simulink model "ComparisonMod1Mod2Thev1Thev2ConstantTorque"  (R2019a)
settings: Solver=ode23t  StartTime=0.0  StopTime=3600  RelTol=1  AbsTol=1e-3  EnableMultiTasking=on
libraries: fl_lib x38, nesl_utility x26, ee_lib x4
settings Model: Creator=nikos  LastModifiedBy=nikos
settings DataIOCC: LimitDataPoints=on  SaveFormat=Array  ReturnWorkspaceOutputs=off
settings OptimizationCC: LifeSpan=inf
settings DebuggingCC: PregeneratedLibrarySubsystemCodeDiagnostic=none  SFUnexpectedBacktrackingDiag=warning  SFNoUnconditionalDefaultTransitionDiag=warning  SFExecutionAtInitializationDiag=none  ArithmeticOperatorsInVariantConditions=warning
settings HardwareCC: ProdBitPerPointer=32  ProdBitPerSizeT=32  ProdBitPerPtrDiffT=32  ProdLargestAtomicFloat=None  ProdIntDivRoundTo=Undefined  ProdEndianess=Unspecified  ProdWordSize=32  ProdHWDeviceType=32-bit Generic
settings ModelReferenceCC: PropagateSignalLabelsOutOfModel=off
settings SFSimCC: SimUseLocalCustomCode=off
settings RTWCC: RTWUseLocalCustomCode=off
settings CodeAppCC: StateflowObjectComments=on
settings GRTTargetCC: TargetLangStandard=C89/C90 (ANSI)  GeneratePreprocessorConditionals=Disable all
settings ConfigComp: CovMetricSettings=dw  CovHtmlReporting=on  CovSaveCumulativeToWorkspaceVar=on  CovSaveSingleToWorkspaceVar=on  CovExternalEMLEnable=off
settings SimscapeCC: SimscapeNormalizeSystem=off  SimscapeLogType=all  SimscapeLogDataHistory=10000

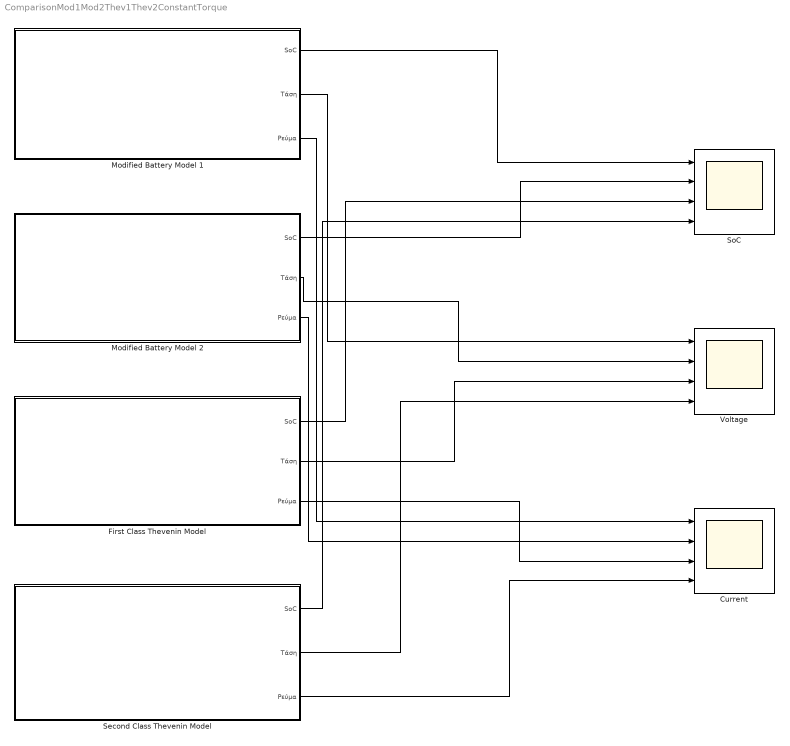
== system ComparisonMod1Mod2Thev1Thev2ConstantTorque ==
  Current : Scope  NumInputPorts=4
  First Class Thevenin Model : Subsystem
  Modified Battery Model 1 : Subsystem
  Modified Battery Model 2 : Subsystem
  "Second Class Thevenin Model " : Subsystem
  SoC : Scope  NumInputPorts=4
  Voltage : Scope  NumInputPorts=4
  wires:
  Modified Battery Model 1/1(SoC) -> SoC/1
  Modified Battery Model 2/1(SoC) -> SoC/2
  First Class Thevenin Model/1("SoC ") -> SoC/3
  "Second Class Thevenin Model "/1("SoC ") -> SoC/4
  Modified Battery Model 1/2(Τάση) -> Voltage/1
  Modified Battery Model 2/2(Τάση) -> Voltage/2
  First Class Thevenin Model/2(Τάση) -> Voltage/3
  "Second Class Thevenin Model "/2(Τάση) -> Voltage/4
  Modified Battery Model 1/3(Ρεύμα) -> Current/1
  Modified Battery Model 2/3(Ρεύμα) -> Current/2
  First Class Thevenin Model/3(Ρεύμα) -> Current/3
  "Second Class Thevenin Model "/3(Ρεύμα) -> Current/4

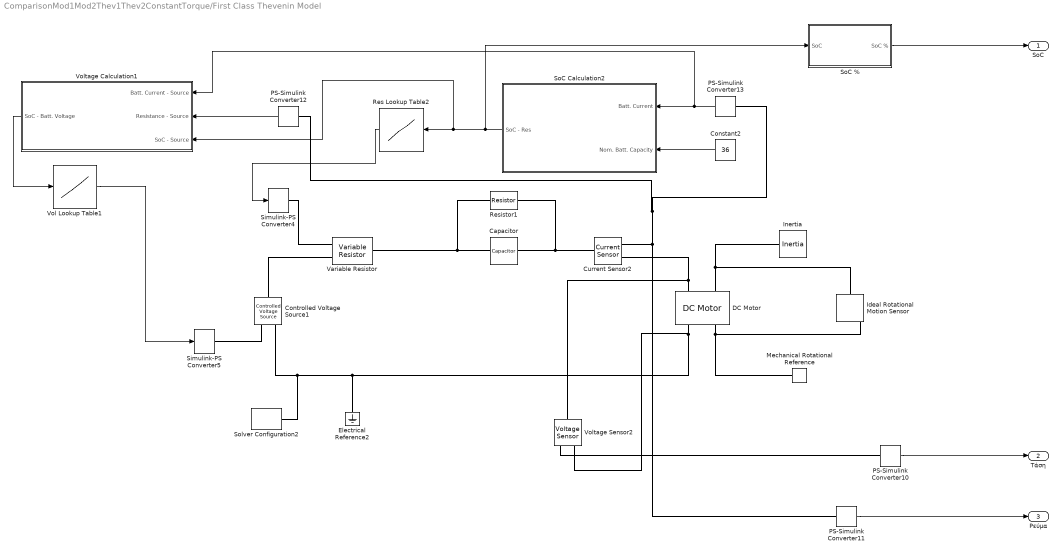
== system ComparisonMod1Mod2Thev1Thev2ConstantTorque/First Class Thevenin Model ==
  Capacitor : fl_lib/Electrical/Electrical Elements/Capacitor  c=1.5 F  r=1e-6 Ohm  g=0 1/Ohm  i_specify=off  i_priority=High  i=0 A  i_nominal_specify=off  i_nominal_unit=A  i_nominal_value=1  v_specify=off  v_priority=High  v=0 V  v_nominal_specify=off  v_nominal_unit=V  v_nominal_value=1  vc_specify=off  vc_priority=High  vc=0 V  vc_nominal_specify=off  vc_nominal_unit=V  vc_nominal_value=1
  Constant2 : Constant  Value=36
  Controlled Voltage Source1 : fl_lib/Electrical/Electrical Sources/Controlled Voltage Source
  Current Sensor2 : fl_lib/Electrical/Electrical Sensors/Current Sensor
  DC Motor : ee_lib/Electromechanical/Brushed Motors/DC Motor  parameterization=2  Ra=3.9 Ohm  La=12e-6 H  emf_or_torque=1  Kv=0.072e-3 V/rpm  Ki=6.876e-4 N*m/A  T_stall=240 mN*m  w_max=4300 rpm  w_rated=15000 rpm  P_rated=0.08 W  V_rated=14.7 V  J=0.01 g*cm^2  lam_param=2  lam=0 N*m/(rad/s)  i_noload=0.16 A  V_i_noload=1.5 V  speed0=0 rpm  alpha=3.93e-3 1/K  Tmeas=25 degC  thermal_mass=100 J/K  initial_temperature=25 degC
      settings: SourceProductName=Simscape Electrical
  Electrical Reference2 : fl_lib/Electrical/Electrical Elements/Electrical Reference
  Ideal Rotational Motion Sensor : fl_lib/Mechanical/Mechanical Sensors/Ideal Rotational Motion Sensor  offset=0 rad
  Inertia : fl_lib/Mechanical/Rotational Elements/Inertia  inertia=0.01 kg*m^2  w_specify=off  w_priority=High  w=0 rad/s  w_nominal_specify=off  w_nominal_unit=rad/s  w_nominal_value=1  t_specify=off  t_priority=None  t=0 N*m  t_nominal_specify=off  t_nominal_unit=N*m  t_nominal_value=1
  Mechanical Rotational Reference : fl_lib/Mechanical/Rotational Elements/Mechanical Rotational Reference
  PS-Simulink Converter{10..13} (4 alike) : nesl_utility/PS-Simulink Converter  PhysicalDomain=network_engine_domain  SubClassName=ps_output  LeftPortType=input  RightPortType=output  PseudoPeriodic=off  Frequencies=[]  Unit=1  AffineConversion=off
  Res Lookup Table2 : Lookup_n-D  NumberOfTableDimensions=1  BreakpointsForDimension1=[0, 10, 20, 30, 40, 50, 60, 70, 80, 90, 100]  Table=[0.011448, 0.011038, 0.011281, 0.011236, 0.010959, 0.010714, 0.010698, 0.010712, 0.010917, 0.011304, 0.011603]  InternalRulePriority=Speed  RndMeth=Simplest  InputSameDT=on
  Resistor1 : fl_lib/Electrical/Electrical Elements/Resistor  R=0.5 Ohm  i_specify=off  i_priority=High  i=0 A  i_nominal_specify=off  i_nominal_unit=A  i_nominal_value=1  v_specify=off  v_priority=High  v=0 V  v_nominal_specify=off  v_nominal_unit=V  v_nominal_value=1
  Simulink-PS Converter4 : nesl_utility/Simulink-PS Converter  PhysicalDomain=network_engine_domain  SubClassName=ps_input  LeftPortType=input  RightPortType=output  PseudoPeriodic=off  Frequencies=[]  NoiseDistribution=none  NoiseParameters=[]  Unit=1  AffineConversion=off  FilteringAndDerivatives=zero  SimscapeFilterOrder=1  InputFilterTimeConstant=0.001  UdotUserProvided=1
  Simulink-PS Converter5 : nesl_utility/Simulink-PS Converter  PhysicalDomain=network_engine_domain  SubClassName=ps_input  LeftPortType=input  RightPortType=output  PseudoPeriodic=off  Frequencies=[]  NoiseDistribution=none  NoiseParameters=[]  Unit=1  AffineConversion=off  FilteringAndDerivatives=filter  SimscapeFilterOrder=1  InputFilterTimeConstant=0.001  UdotUserProvided=1
  SoC % : Subsystem
  SoC Calculation2 : Subsystem
  Solver Configuration2 : nesl_utility/Solver Configuration  PhysicalDomain=network_engine_domain  SubClassName=solver  LeftPortType=input  RightPortType=generic  Tones=[]  Harmonics=[]  SimulateNoise=off  Profile=off  UseLocalSampling=off  EnableSwitchedLinearOptims=on  FrequencyDomain=off  UseCCode=off  RelTol=0.001  AbsTol=1e-06  MinStep=1e-09  ToWorkspace=off  RevertToSquareIcSolve=off  NumHomotopyIterations=100  PhasorMode=off  PhasorModeNumHarmonics=1  DoDC=off  ResidualTolerance=1e-09  UseLocalSolver=off  LocalSolverChoice=NE_BACKWARD_EULER_ADVANCER  LocalSolverSampleTime=0.001  DoFixedCost=off  MaxNonlinIter=3  MaxModeIter=2  LinearAlgebra=Sparse  EquationFormulation=NE_TIME_EF  DelaysMemoryBudget=1024  AutomaticFiltering=on  FilteringTimeConstant=0.001  PartitionStorageMethod=AS_NEEDED  PartitionMemoryBudget=1024  PartitionMethod=FAST
  Variable Resistor : fl_lib/Electrical/Electrical Elements/Variable Resistor  Rmin=0 Ohm  i_specify=off  i_priority=None  i=0 A  i_nominal_specify=off  i_nominal_unit=A  i_nominal_value=1  v_specify=off  v_priority=None  v=0 V  v_nominal_specify=off  v_nominal_unit=V  v_nominal_value=1
  Vol Lookup Table1 : Lookup_n-D  NumberOfTableDimensions=1  BreakpointsForDimension1=[0,10,20,30,40,50,60,70,80,90,100]  Table=[35.042,35.573,36.009,36.393,36.742,37.121,37.937,38.753,39.7,40.821,41.9299999]  InternalRulePriority=Speed  RndMeth=Simplest  InputSameDT=on
  Voltage Calculation1 : Subsystem
  Voltage Sensor2 : fl_lib/Electrical/Electrical Sensors/Voltage Sensor
  "SoC " : Outport
  Τάση : Outport  Port=2
  Ρεύμα : Outport  Port=3
  wires:
  PS-Simulink Converter12/1 -> Voltage Calculation1/2("Resistance - Source ")
  Voltage Calculation1/1("SoC - Batt. Voltage ") -> Vol Lookup Table1/1
  PS-Simulink Converter13/1 -> Voltage Calculation1/1(Batt. Current - Source), SoC Calculation2/1("Batt. Current ")
  PS-Simulink Converter10/1 -> Τάση/1
  Constant2/1 -> SoC Calculation2/2("Nom. Batt. Capacity ")
  SoC Calculation2/1(SoC - Res) -> SoC %/1(SoC), Res Lookup Table2/1, Voltage Calculation1/3(SoC - Source)
  Res Lookup Table2/1 -> Simulink-PS Converter4/1
  Vol Lookup Table1/1 -> Simulink-PS Converter5/1
  PS-Simulink Converter11/1 -> Ρεύμα/1
  SoC %/1(SoC %) -> "SoC "/1
  connections:
  Capacitor/RConn1 -- Resistor1/LConn1 -- Variable Resistor/RConn1
  PS-Simulink Converter13/LConn1 -- PS-Simulink Converter12/LConn1 -- PS-Simulink Converter11/LConn1 -- Current Sensor2/RConn1
  Voltage Sensor2/RConn2 -- DC Motor/RConn1 -- Electrical Reference2/LConn1 -- Controlled Voltage Source1/RConn2 -- Solver Configuration2/RConn1
  Simulink-PS Converter5/RConn1 -- Controlled Voltage Source1/RConn1
  Current Sensor2/RConn2 -- DC Motor/LConn1 -- Voltage Sensor2/LConn1
  Controlled Voltage Source1/LConn1 -- Variable Resistor/LConn2
  Voltage Sensor2/RConn1 -- PS-Simulink Converter10/LConn1
  Simulink-PS Converter4/RConn1 -- Variable Resistor/LConn1
  Capacitor/LConn1 -- Resistor1/RConn1 -- Current Sensor2/LConn1
  Inertia/LConn1 -- Ideal Rotational Motion Sensor/LConn1 -- DC Motor/LConn2
  Mechanical Rotational Reference/LConn1 -- Ideal Rotational Motion Sensor/RConn1 -- DC Motor/RConn2

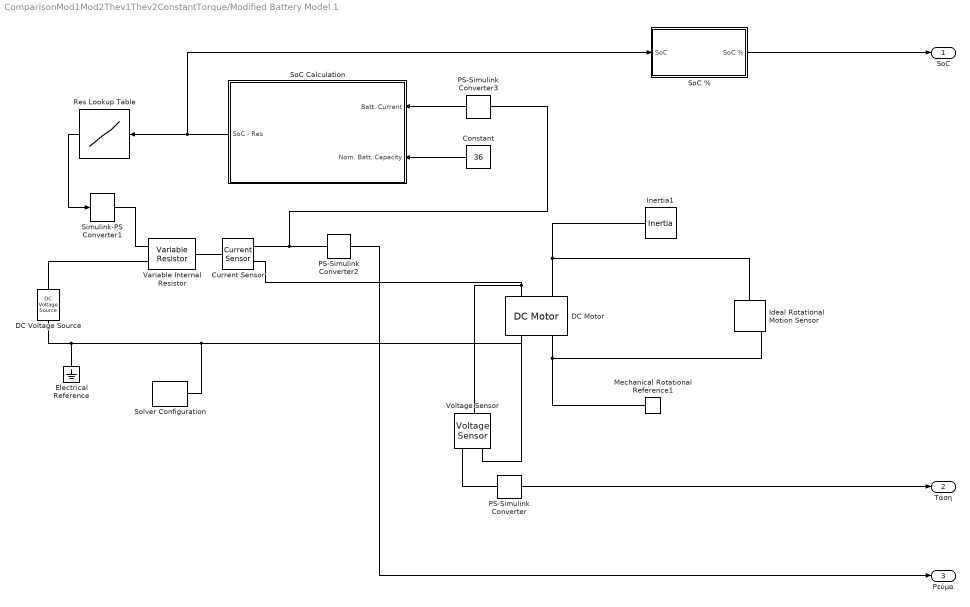
== system ComparisonMod1Mod2Thev1Thev2ConstantTorque/Modified Battery Model 1 ==
  Constant : Constant  Value=36
  Current Sensor : fl_lib/Electrical/Electrical Sensors/Current Sensor
  DC Motor : ee_lib/Electromechanical/Brushed Motors/DC Motor  parameterization=2  Ra=3.9 Ohm  La=12e-6 H  emf_or_torque=1  Kv=0.072e-3 V/rpm  Ki=6.876e-4 N*m/A  T_stall=240 mN*m  w_max=4300 rpm  w_rated=15000 rpm  P_rated=0.08 W  V_rated=14.7 V  J=0.01 g*cm^2  lam_param=2  lam=0 N*m/(rad/s)  i_noload=0.16 A  V_i_noload=1.5 V  speed0=0 rpm  alpha=3.93e-3 1/K  Tmeas=25 degC  thermal_mass=100 J/K  initial_temperature=25 degC
      settings: SourceProductName=Simscape Electrical
  DC Voltage Source : fl_lib/Electrical/Electrical Sources/DC Voltage Source  v0=72 V
  Electrical Reference : fl_lib/Electrical/Electrical Elements/Electrical Reference
  Ideal Rotational Motion Sensor : fl_lib/Mechanical/Mechanical Sensors/Ideal Rotational Motion Sensor  offset=0 rad
  Inertia1 : fl_lib/Mechanical/Rotational Elements/Inertia  inertia=0.01 kg*m^2  w_specify=off  w_priority=High  w=0 rad/s  w_nominal_specify=off  w_nominal_unit=rad/s  w_nominal_value=1  t_specify=off  t_priority=None  t=0 N*m  t_nominal_specify=off  t_nominal_unit=N*m  t_nominal_value=1
  Mechanical Rotational Reference1 : fl_lib/Mechanical/Rotational Elements/Mechanical Rotational Reference
  PS-Simulink Converter : nesl_utility/PS-Simulink Converter  PhysicalDomain=network_engine_domain  SubClassName=ps_output  LeftPortType=input  RightPortType=output  PseudoPeriodic=off  Frequencies=[]  Unit=1  AffineConversion=off
  PS-Simulink Converter2 : nesl_utility/PS-Simulink Converter  PhysicalDomain=network_engine_domain  SubClassName=ps_output  LeftPortType=input  RightPortType=output  PseudoPeriodic=off  Frequencies=[]  Unit=1  AffineConversion=off
  PS-Simulink Converter3 : nesl_utility/PS-Simulink Converter  PhysicalDomain=network_engine_domain  SubClassName=ps_output  LeftPortType=input  RightPortType=output  PseudoPeriodic=off  Frequencies=[]  Unit=1  AffineConversion=off
  Res Lookup Table : Lookup_n-D  NumberOfTableDimensions=1  BreakpointsForDimension1=[0, 10, 20, 30, 40, 50, 60, 70, 80, 90, 100]  Table=[0.011448, 0.011038, 0.011281, 0.011236, 0.010959, 0.010714, 0.010698, 0.010712, 0.010917, 0.011304, 0.011603]  InternalRulePriority=Speed  RndMeth=Simplest  InputSameDT=on
  Simulink-PS Converter1 : nesl_utility/Simulink-PS Converter  PhysicalDomain=network_engine_domain  SubClassName=ps_input  LeftPortType=input  RightPortType=output  PseudoPeriodic=off  Frequencies=[]  NoiseDistribution=none  NoiseParameters=[]  Unit=1  AffineConversion=off  FilteringAndDerivatives=zero  SimscapeFilterOrder=1  InputFilterTimeConstant=0.001  UdotUserProvided=1
  SoC % : Subsystem
  SoC Calculation : Subsystem
  Solver Configuration : nesl_utility/Solver Configuration  PhysicalDomain=network_engine_domain  SubClassName=solver  LeftPortType=input  RightPortType=generic  Tones=[]  Harmonics=[]  SimulateNoise=off  Profile=off  UseLocalSampling=off  EnableSwitchedLinearOptims=on  FrequencyDomain=off  UseCCode=off  RelTol=0.001  AbsTol=1e-06  MinStep=1e-09  ToWorkspace=off  RevertToSquareIcSolve=off  NumHomotopyIterations=100  PhasorMode=off  PhasorModeNumHarmonics=1  DoDC=off  ResidualTolerance=1e-09  UseLocalSolver=off  LocalSolverChoice=NE_BACKWARD_EULER_ADVANCER  LocalSolverSampleTime=0.001  DoFixedCost=off  MaxNonlinIter=3  MaxModeIter=2  LinearAlgebra=Sparse  EquationFormulation=NE_TIME_EF  DelaysMemoryBudget=1024  AutomaticFiltering=on  FilteringTimeConstant=0.001  PartitionStorageMethod=AS_NEEDED  PartitionMemoryBudget=1024  PartitionMethod=FAST
  Variable Internal Resistor : fl_lib/Electrical/Electrical Elements/Variable Resistor  Rmin=1 Ohm  i_specify=off  i_priority=High  i=0 A  i_nominal_specify=off  i_nominal_unit=A  i_nominal_value=1  v_specify=off  v_priority=High  v=0 V  v_nominal_specify=off  v_nominal_unit=V  v_nominal_value=1
  Voltage Sensor : fl_lib/Electrical/Electrical Sensors/Voltage Sensor
  SoC : Outport
  Τάση : Outport  Port=2
  Ρεύμα : Outport  Port=3
  wires:
  SoC Calculation/1(SoC - Res) -> SoC %/1(SoC), Res Lookup Table/1
  PS-Simulink Converter2/1 -> Ρεύμα/1
  Constant/1 -> SoC Calculation/2("Nom. Batt. Capacity ")
  Res Lookup Table/1 -> Simulink-PS Converter1/1
  PS-Simulink Converter3/1 -> SoC Calculation/1("Batt. Current ")
  PS-Simulink Converter/1 -> Τάση/1
  SoC %/1(SoC %) -> SoC/1
  connections:
  PS-Simulink Converter/LConn1 -- Voltage Sensor/RConn1
  Current Sensor/LConn1 -- Variable Internal Resistor/RConn1
  DC Voltage Source/LConn1 -- Variable Internal Resistor/LConn2
  DC Voltage Source/RConn1 -- DC Motor/RConn1 -- Voltage Sensor/RConn2 -- Solver Configuration/RConn1 -- Electrical Reference/LConn1
  Voltage Sensor/LConn1 -- DC Motor/LConn1 -- Current Sensor/RConn2
  PS-Simulink Converter2/LConn1 -- Current Sensor/RConn1 -- PS-Simulink Converter3/LConn1
  Simulink-PS Converter1/RConn1 -- Variable Internal Resistor/LConn1
  DC Motor/LConn2 -- Ideal Rotational Motion Sensor/LConn1 -- Inertia1/LConn1
  DC Motor/RConn2 -- Ideal Rotational Motion Sensor/RConn1 -- Mechanical Rotational Reference1/LConn1

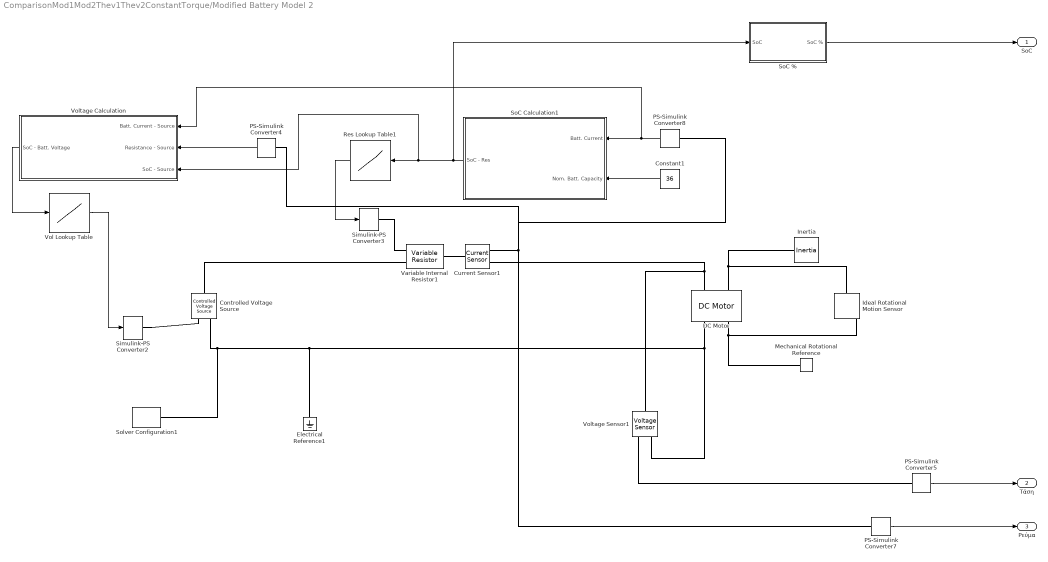
== system ComparisonMod1Mod2Thev1Thev2ConstantTorque/Modified Battery Model 2 ==
  Constant1 : Constant  Value=36
  Controlled Voltage Source : fl_lib/Electrical/Electrical Sources/Controlled Voltage Source
  Current Sensor1 : fl_lib/Electrical/Electrical Sensors/Current Sensor
  DC Motor : ee_lib/Electromechanical/Brushed Motors/DC Motor  parameterization=2  Ra=3.9 Ohm  La=12e-6 H  emf_or_torque=1  Kv=0.072e-3 V/rpm  Ki=6.876e-4 N*m/A  T_stall=240 mN*m  w_max=4300 rpm  w_rated=15000 rpm  P_rated=0.08 W  V_rated=14.7 V  J=0.01 g*cm^2  lam_param=2  lam=0 N*m/(rad/s)  i_noload=0.16 A  V_i_noload=1.5 V  speed0=0 rpm  alpha=3.93e-3 1/K  Tmeas=25 degC  thermal_mass=100 J/K  initial_temperature=25 degC
      settings: SourceProductName=Simscape Electrical
  Electrical Reference1 : fl_lib/Electrical/Electrical Elements/Electrical Reference
  Ideal Rotational Motion Sensor : fl_lib/Mechanical/Mechanical Sensors/Ideal Rotational Motion Sensor  offset=0 rad
  Inertia : fl_lib/Mechanical/Rotational Elements/Inertia  inertia=0.01 kg*m^2  w_specify=off  w_priority=High  w=0 rad/s  w_nominal_specify=off  w_nominal_unit=rad/s  w_nominal_value=1  t_specify=off  t_priority=None  t=0 N*m  t_nominal_specify=off  t_nominal_unit=N*m  t_nominal_value=1
  Mechanical Rotational Reference : fl_lib/Mechanical/Rotational Elements/Mechanical Rotational Reference
  PS-Simulink Converter{4..5,7..8} (4 alike) : nesl_utility/PS-Simulink Converter  PhysicalDomain=network_engine_domain  SubClassName=ps_output  LeftPortType=input  RightPortType=output  PseudoPeriodic=off  Frequencies=[]  Unit=1  AffineConversion=off
  Res Lookup Table1 : Lookup_n-D  NumberOfTableDimensions=1  BreakpointsForDimension1=[0, 10, 20, 30, 40, 50, 60, 70, 80, 90, 100]  Table=[0.011448, 0.011038, 0.011281, 0.011236, 0.010959, 0.010714, 0.010698, 0.010712, 0.010917, 0.011304, 0.011603]  InternalRulePriority=Speed  RndMeth=Simplest  InputSameDT=on
  Simulink-PS Converter2 : nesl_utility/Simulink-PS Converter  PhysicalDomain=network_engine_domain  SubClassName=ps_input  LeftPortType=input  RightPortType=output  PseudoPeriodic=off  Frequencies=[]  NoiseDistribution=none  NoiseParameters=[]  Unit=1  AffineConversion=off  FilteringAndDerivatives=filter  SimscapeFilterOrder=1  InputFilterTimeConstant=0.001  UdotUserProvided=1
  Simulink-PS Converter3 : nesl_utility/Simulink-PS Converter  PhysicalDomain=network_engine_domain  SubClassName=ps_input  LeftPortType=input  RightPortType=output  PseudoPeriodic=off  Frequencies=[]  NoiseDistribution=none  NoiseParameters=[]  Unit=1  AffineConversion=off  FilteringAndDerivatives=zero  SimscapeFilterOrder=1  InputFilterTimeConstant=0.001  UdotUserProvided=1
  SoC % : Subsystem
  SoC Calculation1 : Subsystem
  Solver Configuration1 : nesl_utility/Solver Configuration  PhysicalDomain=network_engine_domain  SubClassName=solver  LeftPortType=input  RightPortType=generic  Tones=[]  Harmonics=[]  SimulateNoise=off  Profile=off  UseLocalSampling=off  EnableSwitchedLinearOptims=on  FrequencyDomain=off  UseCCode=off  RelTol=0.001  AbsTol=1e-06  MinStep=1e-09  ToWorkspace=off  RevertToSquareIcSolve=off  NumHomotopyIterations=100  PhasorMode=off  PhasorModeNumHarmonics=1  DoDC=off  ResidualTolerance=1e-09  UseLocalSolver=off  LocalSolverChoice=NE_BACKWARD_EULER_ADVANCER  LocalSolverSampleTime=0.001  DoFixedCost=off  MaxNonlinIter=3  MaxModeIter=2  LinearAlgebra=Sparse  EquationFormulation=NE_TIME_EF  DelaysMemoryBudget=1024  AutomaticFiltering=on  FilteringTimeConstant=0.001  PartitionStorageMethod=AS_NEEDED  PartitionMemoryBudget=1024  PartitionMethod=FAST
  Variable Internal Resistor1 : fl_lib/Electrical/Electrical Elements/Variable Resistor  Rmin=1 Ohm  i_specify=off  i_priority=High  i=0 A  i_nominal_specify=off  i_nominal_unit=A  i_nominal_value=1  v_specify=off  v_priority=High  v=0 V  v_nominal_specify=off  v_nominal_unit=V  v_nominal_value=1
  Vol Lookup Table : Lookup_n-D  NumberOfTableDimensions=1  BreakpointsForDimension1=[0,10,20,30,40,50,60,70,80,90,100]  Table=[35.042,35.573,36.009,36.393,36.742,37.121,37.937,38.753,39.7,40.821,41.9299999]  InternalRulePriority=Speed  RndMeth=Simplest  InputSameDT=on
  Voltage Calculation : Subsystem
  Voltage Sensor1 : fl_lib/Electrical/Electrical Sensors/Voltage Sensor
  SoC : Outport
  Τάση : Outport  Port=2
  Ρεύμα : Outport  Port=3
  wires:
  Res Lookup Table1/1 -> Simulink-PS Converter3/1
  PS-Simulink Converter5/1 -> Τάση/1
  SoC Calculation1/1(SoC - Res) -> SoC %/1(SoC), Res Lookup Table1/1, Voltage Calculation/3(SoC - Source)
  PS-Simulink Converter8/1 -> SoC Calculation1/1("Batt. Current "), Voltage Calculation/1(Batt. Current - Source)
  PS-Simulink Converter4/1 -> Voltage Calculation/2("Resistance - Source ")
  Constant1/1 -> SoC Calculation1/2("Nom. Batt. Capacity ")
  PS-Simulink Converter7/1 -> Ρεύμα/1
  Voltage Calculation/1("SoC - Batt. Voltage ") -> Vol Lookup Table/1
  Vol Lookup Table/1 -> Simulink-PS Converter2/1
  SoC %/1(SoC %) -> SoC/1
  connections:
  Controlled Voltage Source/RConn2 -- Electrical Reference1/LConn1 -- DC Motor/RConn1 -- Voltage Sensor1/RConn2 -- Solver Configuration1/RConn1
  Current Sensor1/RConn2 -- DC Motor/LConn1 -- Voltage Sensor1/LConn1
  PS-Simulink Converter7/LConn1 -- Current Sensor1/RConn1 -- PS-Simulink Converter8/LConn1 -- PS-Simulink Converter4/LConn1
  Simulink-PS Converter3/RConn1 -- Variable Internal Resistor1/LConn1
  Simulink-PS Converter2/RConn1 -- Controlled Voltage Source/RConn1
  PS-Simulink Converter5/LConn1 -- Voltage Sensor1/RConn1
  Current Sensor1/LConn1 -- Variable Internal Resistor1/RConn1
  Controlled Voltage Source/LConn1 -- Variable Internal Resistor1/LConn2
  DC Motor/LConn2 -- Ideal Rotational Motion Sensor/LConn1 -- Inertia/LConn1
  DC Motor/RConn2 -- Ideal Rotational Motion Sensor/RConn1 -- Mechanical Rotational Reference/LConn1

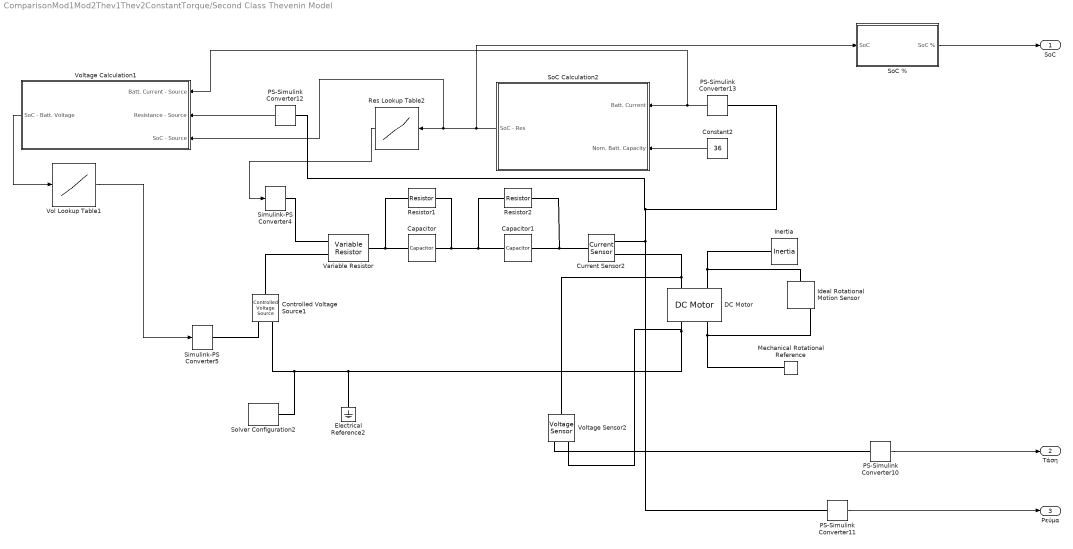
== system ComparisonMod1Mod2Thev1Thev2ConstantTorque/Second Class Thevenin Model  ==
  Capacitor : fl_lib/Electrical/Electrical Elements/Capacitor  c=1.5 F  r=1e-6 Ohm  g=0 1/Ohm  i_specify=off  i_priority=High  i=0 A  i_nominal_specify=off  i_nominal_unit=A  i_nominal_value=1  v_specify=off  v_priority=High  v=0 V  v_nominal_specify=off  v_nominal_unit=V  v_nominal_value=1  vc_specify=off  vc_priority=High  vc=0 V  vc_nominal_specify=off  vc_nominal_unit=V  vc_nominal_value=1
  Capacitor1 : fl_lib/Electrical/Electrical Elements/Capacitor  c=1.5 F  r=1e-6 Ohm  g=0 1/Ohm  i_specify=off  i_priority=High  i=0 A  i_nominal_specify=off  i_nominal_unit=A  i_nominal_value=1  v_specify=off  v_priority=High  v=0 V  v_nominal_specify=off  v_nominal_unit=V  v_nominal_value=1  vc_specify=off  vc_priority=High  vc=0 V  vc_nominal_specify=off  vc_nominal_unit=V  vc_nominal_value=1
  Constant2 : Constant  Value=36
  Controlled Voltage Source1 : fl_lib/Electrical/Electrical Sources/Controlled Voltage Source
  Current Sensor2 : fl_lib/Electrical/Electrical Sensors/Current Sensor
  DC Motor : ee_lib/Electromechanical/Brushed Motors/DC Motor  parameterization=2  Ra=3.9 Ohm  La=12e-6 H  emf_or_torque=1  Kv=0.072e-3 V/rpm  Ki=6.876e-4 N*m/A  T_stall=240 mN*m  w_max=4300 rpm  w_rated=15000 rpm  P_rated=0.08 W  V_rated=14.7 V  J=0.01 g*cm^2  lam_param=2  lam=0 N*m/(rad/s)  i_noload=0.16 A  V_i_noload=1.5 V  speed0=0 rpm  alpha=3.93e-3 1/K  Tmeas=25 degC  thermal_mass=100 J/K  initial_temperature=25 degC
      settings: SourceProductName=Simscape Electrical
  Electrical Reference2 : fl_lib/Electrical/Electrical Elements/Electrical Reference
  Ideal Rotational Motion Sensor : fl_lib/Mechanical/Mechanical Sensors/Ideal Rotational Motion Sensor  offset=0 rad
  Inertia : fl_lib/Mechanical/Rotational Elements/Inertia  inertia=0.01 kg*m^2  w_specify=off  w_priority=High  w=0 rad/s  w_nominal_specify=off  w_nominal_unit=rad/s  w_nominal_value=1  t_specify=off  t_priority=None  t=0 N*m  t_nominal_specify=off  t_nominal_unit=N*m  t_nominal_value=1
  Mechanical Rotational Reference : fl_lib/Mechanical/Rotational Elements/Mechanical Rotational Reference
  PS-Simulink Converter{10..13} (4 alike) : nesl_utility/PS-Simulink Converter  PhysicalDomain=network_engine_domain  SubClassName=ps_output  LeftPortType=input  RightPortType=output  PseudoPeriodic=off  Frequencies=[]  Unit=1  AffineConversion=off
  Res Lookup Table2 : Lookup_n-D  NumberOfTableDimensions=1  BreakpointsForDimension1=[0, 10, 20, 30, 40, 50, 60, 70, 80, 90, 100]  Table=[0.011448, 0.011038, 0.011281, 0.011236, 0.010959, 0.010714, 0.010698, 0.010712, 0.010917, 0.011304, 0.011603]  InternalRulePriority=Speed  RndMeth=Simplest  InputSameDT=on
  Resistor1 : fl_lib/Electrical/Electrical Elements/Resistor  R=0.5 Ohm  i_specify=off  i_priority=High  i=0 A  i_nominal_specify=off  i_nominal_unit=A  i_nominal_value=1  v_specify=off  v_priority=High  v=0 V  v_nominal_specify=off  v_nominal_unit=V  v_nominal_value=1
  Resistor2 : fl_lib/Electrical/Electrical Elements/Resistor  R=0.5 Ohm  i_specify=off  i_priority=High  i=0 A  i_nominal_specify=off  i_nominal_unit=A  i_nominal_value=1  v_specify=off  v_priority=High  v=0 V  v_nominal_specify=off  v_nominal_unit=V  v_nominal_value=1
  Simulink-PS Converter4 : nesl_utility/Simulink-PS Converter  PhysicalDomain=network_engine_domain  SubClassName=ps_input  LeftPortType=input  RightPortType=output  PseudoPeriodic=off  Frequencies=[]  NoiseDistribution=none  NoiseParameters=[]  Unit=1  AffineConversion=off  FilteringAndDerivatives=zero  SimscapeFilterOrder=1  InputFilterTimeConstant=0.001  UdotUserProvided=1
  Simulink-PS Converter5 : nesl_utility/Simulink-PS Converter  PhysicalDomain=network_engine_domain  SubClassName=ps_input  LeftPortType=input  RightPortType=output  PseudoPeriodic=off  Frequencies=[]  NoiseDistribution=none  NoiseParameters=[]  Unit=1  AffineConversion=off  FilteringAndDerivatives=filter  SimscapeFilterOrder=1  InputFilterTimeConstant=0.001  UdotUserProvided=1
  SoC % : Subsystem
  SoC Calculation2 : Subsystem
  Solver Configuration2 : nesl_utility/Solver Configuration  PhysicalDomain=network_engine_domain  SubClassName=solver  LeftPortType=input  RightPortType=generic  Tones=[]  Harmonics=[]  SimulateNoise=off  Profile=off  UseLocalSampling=off  EnableSwitchedLinearOptims=on  FrequencyDomain=off  UseCCode=off  RelTol=0.001  AbsTol=1e-06  MinStep=1e-09  ToWorkspace=off  RevertToSquareIcSolve=off  NumHomotopyIterations=100  PhasorMode=off  PhasorModeNumHarmonics=1  DoDC=off  ResidualTolerance=1e-09  UseLocalSolver=off  LocalSolverChoice=NE_BACKWARD_EULER_ADVANCER  LocalSolverSampleTime=0.001  DoFixedCost=off  MaxNonlinIter=3  MaxModeIter=2  LinearAlgebra=Sparse  EquationFormulation=NE_TIME_EF  DelaysMemoryBudget=1024  AutomaticFiltering=on  FilteringTimeConstant=0.001  PartitionStorageMethod=AS_NEEDED  PartitionMemoryBudget=1024  PartitionMethod=FAST
  Variable Resistor : fl_lib/Electrical/Electrical Elements/Variable Resistor  Rmin=0 Ohm  i_specify=off  i_priority=None  i=0 A  i_nominal_specify=off  i_nominal_unit=A  i_nominal_value=1  v_specify=off  v_priority=None  v=0 V  v_nominal_specify=off  v_nominal_unit=V  v_nominal_value=1
  Vol Lookup Table1 : Lookup_n-D  NumberOfTableDimensions=1  BreakpointsForDimension1=[0,10,20,30,40,50,60,70,80,90,100]  Table=[35.042,35.573,36.009,36.393,36.742,37.121,37.937,38.753,39.7,40.821,41.9299999]  InternalRulePriority=Speed  RndMeth=Simplest  InputSameDT=on
  Voltage Calculation1 : Subsystem
  Voltage Sensor2 : fl_lib/Electrical/Electrical Sensors/Voltage Sensor
  "SoC " : Outport
  Τάση : Outport  Port=2
  Ρεύμα : Outport  Port=3
  wires:
  PS-Simulink Converter13/1 -> Voltage Calculation1/1(Batt. Current - Source), SoC Calculation2/1("Batt. Current ")
  SoC Calculation2/1(SoC - Res) -> SoC %/1(SoC), Res Lookup Table2/1, Voltage Calculation1/3(SoC - Source)
  PS-Simulink Converter11/1 -> Ρεύμα/1
  PS-Simulink Converter12/1 -> Voltage Calculation1/2("Resistance - Source ")
  PS-Simulink Converter10/1 -> Τάση/1
  Constant2/1 -> SoC Calculation2/2("Nom. Batt. Capacity ")
  Res Lookup Table2/1 -> Simulink-PS Converter4/1
  Vol Lookup Table1/1 -> Simulink-PS Converter5/1
  Voltage Calculation1/1("SoC - Batt. Voltage ") -> Vol Lookup Table1/1
  SoC %/1(SoC %) -> "SoC "/1
  connections:
  Voltage Sensor2/RConn1 -- PS-Simulink Converter10/LConn1
  Controlled Voltage Source1/LConn1 -- Variable Resistor/LConn2
  Capacitor/LConn1 -- Resistor2/LConn1 -- Capacitor1/RConn1 -- Resistor1/RConn1
  Solver Configuration2/RConn1 -- Voltage Sensor2/RConn2 -- DC Motor/RConn1 -- Electrical Reference2/LConn1 -- Controlled Voltage Source1/RConn2
  Simulink-PS Converter5/RConn1 -- Controlled Voltage Source1/RConn1
  Capacitor1/LConn1 -- Resistor2/RConn1 -- Current Sensor2/LConn1
  Current Sensor2/RConn2 -- DC Motor/LConn1 -- Voltage Sensor2/LConn1
  PS-Simulink Converter13/LConn1 -- PS-Simulink Converter11/LConn1 -- Current Sensor2/RConn1 -- PS-Simulink Converter12/LConn1
  Capacitor/RConn1 -- Resistor1/LConn1 -- Variable Resistor/RConn1
  Simulink-PS Converter4/RConn1 -- Variable Resistor/LConn1
  Inertia/LConn1 -- Ideal Rotational Motion Sensor/LConn1 -- DC Motor/LConn2
  Mechanical Rotational Reference/LConn1 -- Ideal Rotational Motion Sensor/RConn1 -- DC Motor/RConn2

== system ComparisonMod1Mod2Thev1Thev2ConstantTorque/First Class Thevenin Model/SoC % ==
  SoC : Inport
  Gain : Gain  Gain=1/36
  Gain1 : Gain  Gain=100
  SoC % : Outport
  wires:
  Gain/1 -> Gain1/1
  SoC/1 -> Gain/1
  Gain1/1 -> SoC %/1

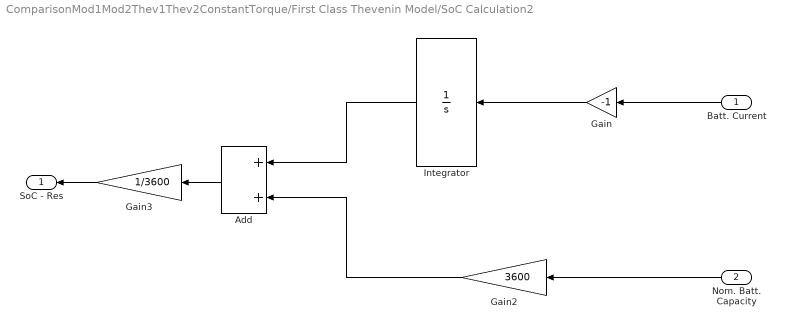
== system ComparisonMod1Mod2Thev1Thev2ConstantTorque/First Class Thevenin Model/SoC Calculation2 ==
  "Batt. Current " : Inport
  "Nom. Batt. Capacity " : Inport  Port=2  OutMin=0  OutMax=100
  Add : Sum
  Gain : Gain  Gain=-1
  Gain2 : Gain  Gain=3600
  Gain3 : Gain  Gain=1/3600
  Integrator : Integrator
  SoC - Res : Outport
  wires:
  Gain3/1 -> SoC - Res/1
  Integrator/1 -> Add/1
  Add/1 -> Gain3/1
  Gain2/1 -> Add/2
  "Nom. Batt. Capacity "/1 -> Gain2/1
  Gain/1 -> Integrator/1
  "Batt. Current "/1 -> Gain/1

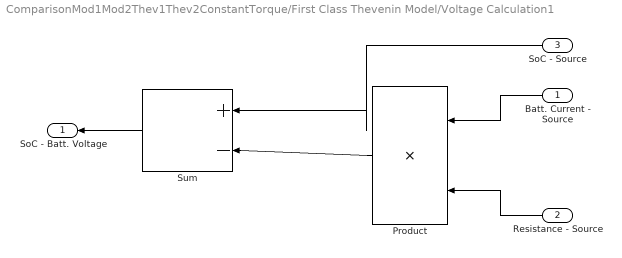
== system ComparisonMod1Mod2Thev1Thev2ConstantTorque/First Class Thevenin Model/Voltage Calculation1 ==
  Batt. Current - Source : Inport
  "Resistance - Source " : Inport  Port=2
  SoC - Source : Inport  Port=3
  Product : Product
  Sum : Sum  Inputs=|+-
  "SoC - Batt. Voltage " : Outport
  wires:
  Product/1 -> Sum/2
  Batt. Current - Source/1 -> Product/1
  "Resistance - Source "/1 -> Product/2
  SoC - Source/1 -> Sum/1
  Sum/1 -> "SoC - Batt. Voltage "/1

== system ComparisonMod1Mod2Thev1Thev2ConstantTorque/Modified Battery Model 1/SoC % ==
  SoC : Inport
  Gain : Gain  Gain=1/36
  Gain1 : Gain  Gain=100
  SoC % : Outport
  wires:
  Gain/1 -> Gain1/1
  SoC/1 -> Gain/1
  Gain1/1 -> SoC %/1

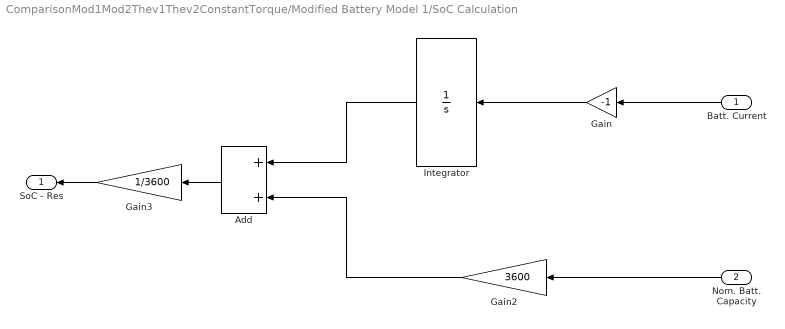
== system ComparisonMod1Mod2Thev1Thev2ConstantTorque/Modified Battery Model 1/SoC Calculation ==
  "Batt. Current " : Inport
  "Nom. Batt. Capacity " : Inport  Port=2  OutMin=0  OutMax=100
  Add : Sum
  Gain : Gain  Gain=-1
  Gain2 : Gain  Gain=3600
  Gain3 : Gain  Gain=1/3600
  Integrator : Integrator
  SoC - Res : Outport
  wires:
  "Batt. Current "/1 -> Gain/1
  Gain/1 -> Integrator/1
  "Nom. Batt. Capacity "/1 -> Gain2/1
  Gain2/1 -> Add/2
  Add/1 -> Gain3/1
  Integrator/1 -> Add/1
  Gain3/1 -> SoC - Res/1

== system ComparisonMod1Mod2Thev1Thev2ConstantTorque/Modified Battery Model 2/SoC % ==
  SoC : Inport
  Gain : Gain  Gain=1/36
  Gain1 : Gain  Gain=100
  SoC % : Outport
  wires:
  Gain/1 -> Gain1/1
  SoC/1 -> Gain/1
  Gain1/1 -> SoC %/1

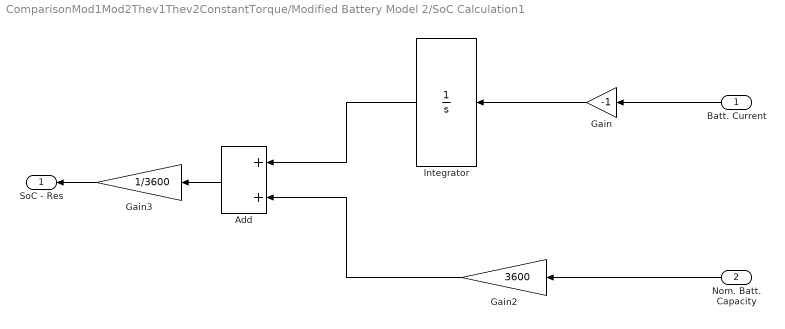
== system ComparisonMod1Mod2Thev1Thev2ConstantTorque/Modified Battery Model 2/SoC Calculation1 ==
  "Batt. Current " : Inport
  "Nom. Batt. Capacity " : Inport  Port=2  OutMin=0  OutMax=100
  Add : Sum
  Gain : Gain  Gain=-1
  Gain2 : Gain  Gain=3600
  Gain3 : Gain  Gain=1/3600
  Integrator : Integrator
  SoC - Res : Outport
  wires:
  "Batt. Current "/1 -> Gain/1
  Gain/1 -> Integrator/1
  "Nom. Batt. Capacity "/1 -> Gain2/1
  Gain2/1 -> Add/2
  Add/1 -> Gain3/1
  Integrator/1 -> Add/1
  Gain3/1 -> SoC - Res/1

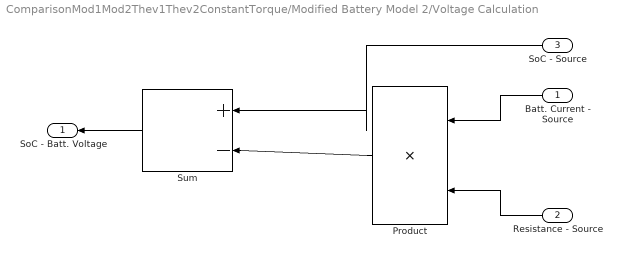
== system ComparisonMod1Mod2Thev1Thev2ConstantTorque/Modified Battery Model 2/Voltage Calculation ==
  Batt. Current - Source : Inport
  "Resistance - Source " : Inport  Port=2
  SoC - Source : Inport  Port=3
  Product : Product
  Sum : Sum  Inputs=|+-
  "SoC - Batt. Voltage " : Outport
  wires:
  Sum/1 -> "SoC - Batt. Voltage "/1
  SoC - Source/1 -> Sum/1
  "Resistance - Source "/1 -> Product/2
  Batt. Current - Source/1 -> Product/1
  Product/1 -> Sum/2

== system ComparisonMod1Mod2Thev1Thev2ConstantTorque/Second Class Thevenin Model /SoC % ==
  SoC : Inport
  Gain : Gain  Gain=1/36
  Gain1 : Gain  Gain=100
  SoC % : Outport
  wires:
  Gain/1 -> Gain1/1
  SoC/1 -> Gain/1
  Gain1/1 -> SoC %/1

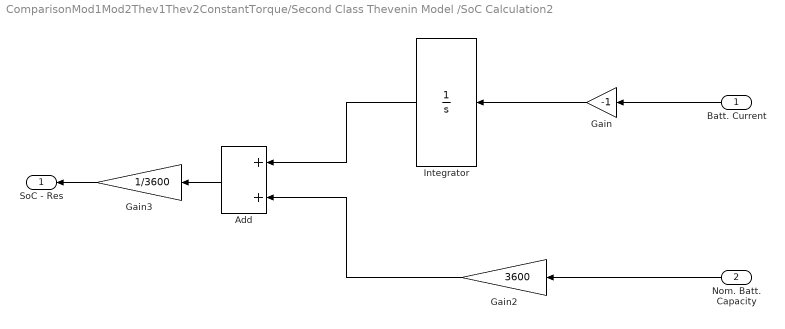
== system ComparisonMod1Mod2Thev1Thev2ConstantTorque/Second Class Thevenin Model /SoC Calculation2 ==
  "Batt. Current " : Inport
  "Nom. Batt. Capacity " : Inport  Port=2  OutMin=0  OutMax=100
  Add : Sum
  Gain : Gain  Gain=-1
  Gain2 : Gain  Gain=3600
  Gain3 : Gain  Gain=1/3600
  Integrator : Integrator
  SoC - Res : Outport
  wires:
  Gain3/1 -> SoC - Res/1
  Integrator/1 -> Add/1
  Add/1 -> Gain3/1
  Gain2/1 -> Add/2
  "Nom. Batt. Capacity "/1 -> Gain2/1
  Gain/1 -> Integrator/1
  "Batt. Current "/1 -> Gain/1

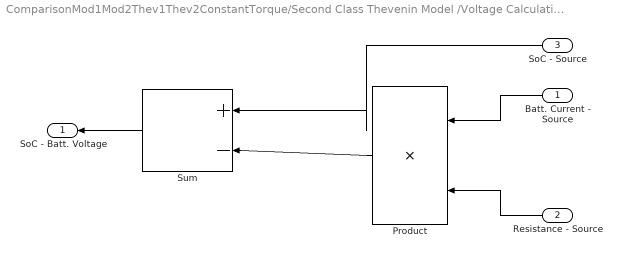
== system ComparisonMod1Mod2Thev1Thev2ConstantTorque/Second Class Thevenin Model /Voltage Calculation1 ==
  Batt. Current - Source : Inport
  "Resistance - Source " : Inport  Port=2
  SoC - Source : Inport  Port=3
  Product : Product
  Sum : Sum  Inputs=|+-
  "SoC - Batt. Voltage " : Outport
  wires:
  Product/1 -> Sum/2
  Batt. Current - Source/1 -> Product/1
  "Resistance - Source "/1 -> Product/2
  SoC - Source/1 -> Sum/1
  Sum/1 -> "SoC - Batt. Voltage "/1
